simulink model "final_quadruped_210522"  (R2021a)
settings: Solver=ode15s  StartTime=0.0  StopTime=2  RelTol=1e-6  EnableMultiTasking=on
values from neighbouring files (symbols this model uses):
  foot_x = 8    [bipedparameters.m]    (also in fcn.m; finalrobotParameters.m; finalrobotParameters_110522.m; finalrobotParameters_140522.m)
  foot_y = 6    [bipedparameters.m]    (also in fcn.m; finalrobotParameters.m; finalrobotParameters_110522.m; finalrobotParameters_140522.m)
  foot_z = 1    [bipedparameters.m]    (also in fcn.m; finalrobotParameters.m; finalrobotParameters_110522.m; finalrobotParameters_140522.m)
  height_plane = 0.025    [bipedparameters.m]    (also in finalrobotParameters.m; finalrobotParameters_110522.m; finalrobotParameters_140522.m; finalrobotParameters_240522.m)
  kd = 1000    [bipedparameters.m]    (also in finalrobotParameters_140522.m = 5; finalrobotParameters_240522.m)
  ki = 1000    [bipedparameters.m]    (also in finalrobotParameters_140522.m = 5; finalrobotParameters_240522.m)
  kp = 1000    [bipedparameters.m]    (also in finalrobotParameters_140522.m = 5; finalrobotParameters_240522.m)
  lower_leg_length = 10    [bipedparameters.m]    (also in fcn.m; finalrobotParameters.m; finalrobotParameters_110522.m; finalrobotParameters_140522.m)
  m_ll = density*leg_radius*leg_radius*lower_leg_length*3.141592653589*0.01*0.01*0.01    (= 0.0176714586764)    [bipedparameters.m]    (also in fcn.m; finalrobotParameters_140522.m; finalrobotParameters_240522.m; hdotlb.m)
  m_ul = density*leg_radius*leg_radius*upper_leg_length*3.141592653589*0.01*0.01*0.01    (= 0.0176714586764)    [bipedparameters.m]    (also in fcn.m; finalrobotParameters_140522.m; finalrobotParameters_240522.m; hdotlb.m)
  plane_x = 25    [bipedparameters.m]    (also in finalrobotParameters.m; finalrobotParameters_110522.m; finalrobotParameters_140522.m; finalrobotParameters_240522.m)
  plane_y = 3    [bipedparameters.m]    (also in finalrobotParameters.m; finalrobotParameters_110522.m; finalrobotParameters_140522.m; finalrobotParameters_240522.m)
  torso_offset_x = -0.5    [bipedparameters.m]    (also in finalrobotParameters.m = 10; finalrobotParameters_110522.m = 10; finalrobotParameters_140522.m = 10; finalrobotParameters_240522.m = 10)
  torso_offset_z = -2    [bipedparameters.m]    (also in finalrobotParameters.m; finalrobotParameters_110522.m; finalrobotParameters_140522.m; finalrobotParameters_240522.m)
  torso_x = 5    [bipedparameters.m]    (also in fcn.m = 25; finalrobotParameters.m = 25; finalrobotParameters_110522.m = 25; finalrobotParameters_140522.m = 25)
  torso_y = 10    [bipedparameters.m]    (also in fcn.m = 16; finalrobotParameters.m = 16; finalrobotParameters_110522.m = 16; finalrobotParameters_140522.m = 16)
  torso_z = 8    [bipedparameters.m]    (also in fcn.m = 10; finalrobotParameters.m = 10; finalrobotParameters_110522.m = 10; finalrobotParameters_140522.m = 10)
  upper_leg_length = 10    [bipedparameters.m]    (also in fcn.m; finalrobotParameters.m; finalrobotParameters_110522.m; finalrobotParameters_140522.m)
undefined symbols (not defined in the file or in its folder): X, Y, Z
libraries: nesl_utility x151, sm_lib x71, Contact_Forces_Lib x16, pid_lib x12, fl_lib x4
(part 6 of 7)

== system final_quadruped_210522/Model/Right Leg Back/Knee ==
  note: accelerationRBknee
  note: Meas for knee
  tddRB_knee : Inport
  t2ddknee : Inport  Port=2
  Bus Creator : BusCreator  Inputs=3
  Knee joint : sm_lib/Joints/Revolute Joint  JointMode=Normal  SenseConstraintForce=off  SenseConstraintForceX=off  SenseConstraintForceY=off  SenseConstraintForceZ=off  SenseConstraintTorque=off  SenseConstraintTorqueX=off  SenseConstraintTorqueY=off  SenseConstraintTorqueZ=off  SenseTotalForce=off  SenseTotalForceX=off  SenseTotalForceY=off  SenseTotalForceZ=off  SenseTotalTorque=off  SenseTotalTorqueX=off  SenseTotalTorqueY=off  SenseTotalTorqueZ=off  CompositeWrenchDir=FollowerOnBase  CompositeWrenchFrame=BaseFrame  EquilibriumPosition=0  EquilibriumPositionUnits=deg  SpringStiffness=0  SpringStiffnessUnits=N*m/deg  DampingCoefficient=0  DampingCoefficientUnits=N*m/(deg/s)  TorqueActuationMode=InputTorque  MotionActuationMode=ComputedMotion  SensePosition=on  SenseVelocity=on  SenseAcceleration=on  SenseTorqueForce=off  SenseLowerLimitTorqueForce=off  SenseUpperLimitTorqueForce=off  LowerLimitSpecify=on  LowerLimitBound=0  LowerLimitBoundUnits=deg  LowerLimitStiffness=1e4  LowerLimitStiffnessUnits=N*m/deg  LowerLimitDamping=10  LowerLimitDampingUnits=N*m/(deg/s)  LowerLimitTransitionRegionWidth=0.1  LowerLimitTransitionRegionWidthUnits=deg  UpperLimitSpecify=on  UpperLimitBound=20  UpperLimitBoundUnits=deg  UpperLimitStiffness=1e4  UpperLimitStiffnessUnits=N*m/deg  UpperLimitDamping=10  UpperLimitDampingUnits=N*m/(deg/s)  UpperLimitTransitionRegionWidth=0.1  UpperLimitTransitionRegionWidthUnits=deg  PositionTargetSpecify=off  PositionTargetPriority=High  PositionTargetValue=0  PositionTargetValueUnits=deg  VelocityTargetSpecify=off  VelocityTargetPriority=High  VelocityTargetValue=0  VelocityTargetValueUnits=deg/s
  PID Controller : pid_lib/PID Controller  Controller=PID  Form=Parallel  TimeDomain=Continuous-time  UseExternalTs=off  SampleTime=-1  IntegratorMethod=Forward Euler  FilterMethod=Forward Euler  ControllerParametersSource=internal  P=kp  I=ki  D=kd  UseFilter=on  N=100  TunerSelectOption=Transfer Function Based (PID Tuner App)  InitialConditionSource=internal  InitialConditionForIntegrator=0  InitialConditionForFilter=0  DifferentiatorICPrevScaledInput=0  ExternalReset=none  TrackingMode=off  Kt=1  LimitOutput=off  SatLimitsSource=internal  UpperSaturationLimit=inf  LowerSaturationLimit=-inf  LinearizeAsGain=on  AntiWindupMode=none  Kb=1  POutMin=[]  POutMax=[]  IOutMin=[]  IOutMax=[]  DOutMin=[]  DOutMax=[]  NOutMin=[]  NOutMax=[]  SumOutMin=[]  SumOutMax=[]  SaturationOutMin=[]  SaturationOutMax=[]  PParamMin=[]  PParamMax=[]  IParamMin=[]  IParamMax=[]  DParamMin=[]  DParamMax=[]  NParamMin=[]  NParamMax=[]  KbParamMin=[]  KbParamMax=[]  KtParamMin=[]  KtParamMax=[]  KbOutMin=[]  KbOutMax=[]  KtOutMin=[]  KtOutMax=[]  IntegratorOutMin=[]  IntegratorOutMax=[]  FilterOutMin=[]  FilterOutMax=[]  SumI1OutMin=[]  SumI1OutMax=[]  SumI2OutMin=[]  SumI2OutMax=[]  SumI3OutMin=[]  SumI3OutMax=[]  SumI4OutMin=[]  SumI4OutMax=[]  SumDOutMin=[]  SumDOutMax=[]  DifferentiatorOutMin=[]  DifferentiatorOutMax=[]  FilterDiffOutCoefMin=[]  FilterDiffOutCoefMax=[]  ReciprocalOutMin=[]  ReciprocalOutMax=[]  SumDenOutMin=[]  SumDenOutMax=[]  SumNumOutMin=[]  SumNumOutMax=[]  DivideOutMin=[]  DivideOutMax=[]  UdiffTsProdOutMin=[]  UdiffTsProdOutMax=[]  NTsProdOutMin=[]  NTsProdOutMax=[]  UintegralTsProdOutMin=[]  UintegralTsProdOutMax=[]  UngainTsProdOutMin=[]  UngainTsProdOutMax=[]  IntegratorContinuousStateAttributes=''  IntegratorStateMustResolveToSignalObject=off  IntegratorRTWStateStorageClass=Auto  FilterContinuousStateAttributes=''  FilterStateMustResolveToSignalObject=off  FilterRTWStateStorageClass=Auto  ParallelPVariant=InternalParameters  IdealPVariant=Disabled  IVariant=InternalParameters  DVariant=InternalParameters  IntegratorVariant=Continuous  SatVariant=Disabled  AWVariant=Passthrough  PCopyVariant=Disabled  TRVariant=Disabled  FdbkBlocksVariant=Forward  IdealPFdbkVariant=Disabled  SatFdbkVariant=Disabled  DerivativeFilterVariant=ContFilter  NVariant=InternalParameters  NCopyVariant=Disabled  FilterICVariant=InternalICsFilter  IntegratorICVariant=InternalICs  ExternalResetVariant=Disabled  TRSumVariant=Passthrough  SumFdbkVariant=Disabled  SumVariant=Sum_PID  TsampFilterVariant=InternalTs  TsampNgainVariant=Passthrough  TsampIntegralVariant=Passthrough  ExternalSaturationOutDataTypeStr=Inherit: Same as second input
  PS-Simulink Converter : nesl_utility/PS-Simulink Converter  PhysicalDomain=network_engine_domain  SubClassName=ps_output  LeftPortType=input  RightPortType=output  PseudoPeriodic=off  Frequencies=[]  Unit=inherit  AffineConversion=off
      settings: SourceProductBaseCode=PW,SS
  PS-Simulink Converter1 : nesl_utility/PS-Simulink Converter  PhysicalDomain=network_engine_domain  SubClassName=ps_output  LeftPortType=input  RightPortType=output  PseudoPeriodic=off  Frequencies=[]  Unit=1  AffineConversion=off
      settings: SourceProductBaseCode=PW,SS
  PS-Simulink Converter3 : nesl_utility/PS-Simulink Converter  PhysicalDomain=network_engine_domain  SubClassName=ps_output  LeftPortType=input  RightPortType=output  PseudoPeriodic=off  Frequencies=[]  Unit=1  AffineConversion=off
      settings: SourceProductBaseCode=PW,SS
  Scope : Scope
  Scope1 : Scope
  Scope2 : Scope
  Simulink-PS Converter : nesl_utility/Simulink-PS Converter  PhysicalDomain=network_engine_domain  SubClassName=ps_input  LeftPortType=input  RightPortType=output  PseudoPeriodic=off  Frequencies=[]  NoiseDistribution=none  NoiseParameters=[]  Unit=1  AffineConversion=off  FilteringAndDerivatives=provide  SimscapeFilterOrder=1  InputFilterTimeConstant=0.001  UdotUserProvided=0
      settings: SourceProductBaseCode=PW,SS
  Sum : Sum  Inputs=|+-
  Conn1 : PMIOPort  Side=Left
  Conn2 : PMIOPort  Port=2  Side=Right
  q : PMIOPort  Port=3  Side=Left
  meas : Outport
  Outport : Outport  Port=2
  Outport1 : Outport  Port=3
  wires:
  Bus Creator/1 -> meas/1
  PS-Simulink Converter3/1 -> Bus Creator/1  "angleRBknee"
  Sum/1 -> Scope/1, PID Controller/1
  PS-Simulink Converter1/1 -> Outport/1, Bus Creator/2  "speedRBknee"
  PID Controller/1 -> Bus Creator/3, Simulink-PS Converter/1, Scope1/1  "torqueRBknee"
  tddRB_knee/1 -> Scope2/1
  t2ddknee/1 -> Sum/1
  PS-Simulink Converter/1 -> Outport1/1, Sum/2
  connections:
  Conn2/RConn1 -- Knee joint/RConn1
  q/RConn1 -- PS-Simulink Converter3/LConn1 -- Knee joint/RConn2
  Knee joint/LConn1 -- Conn1/RConn1
  Knee joint/RConn3 -- PS-Simulink Converter1/LConn1
  Simulink-PS Converter/RConn1 -- Knee joint/LConn2
  Knee joint/RConn4 -- PS-Simulink Converter/LConn1

== system final_quadruped_210522/Model/Right Leg Back/Measuring Component ==
  Fn : Inport
  Hip : Inport  Port=2
  Fr : Inport  Port=3
  Knee : Inport  Port=4
  Ankle : Inport  Port=5
  Bus Creator : BusCreator  Inputs=9
  Bus Selector : BusSelector  OutputSignals=angleRBknee,speedRBknee,torqueRBknee
  Bus Selector1 : BusSelector  OutputSignals=angleRBhip,speedRBhip,torqueRBhip
  Meas : Outport  VectorParamsAs1DForOutWhenUnconnected=off
  wires:
  Ankle/1 -> Bus Creator/3
  Bus Selector1/2 -> Bus Creator/8  "<speedRBhip>"
  Hip/1 -> Bus Selector1/1
  Fn/1 -> Bus Creator/1
  Bus Selector/3 -> Bus Creator/6  "<torqueRBknee>"
  Bus Creator/1 -> Meas/1
  Fr/1 -> Bus Creator/2
  Knee/1 -> Bus Selector/1
  Bus Selector1/3 -> Bus Creator/9  "<torqueRBhip>"
  Bus Selector/2 -> Bus Creator/5  "<speedRBknee>"
  Bus Selector/1 -> Bus Creator/4  "<angleRBknee>"
  Bus Selector1/1 -> Bus Creator/7  "<angleRBhip>"

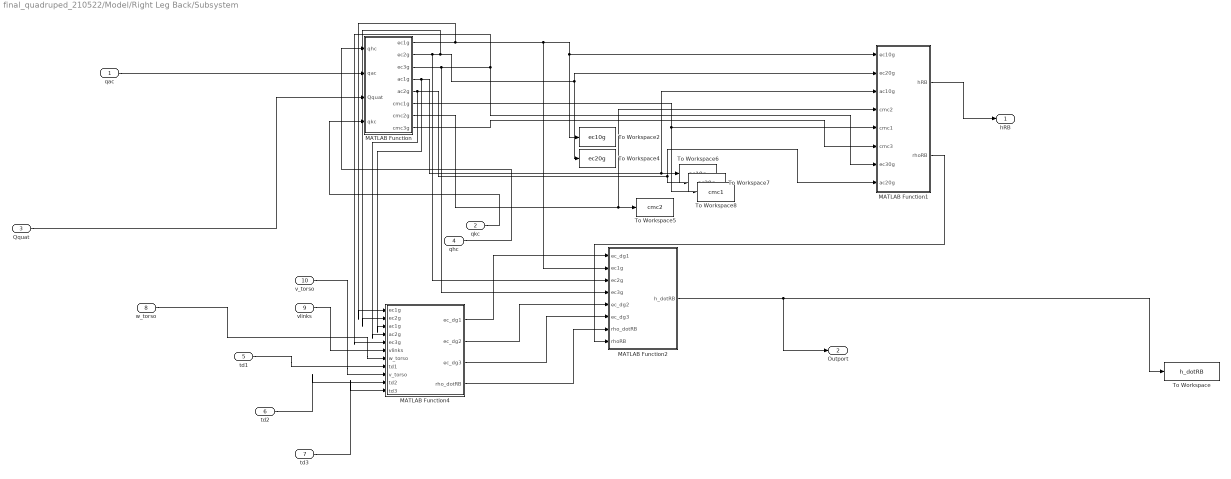
== system final_quadruped_210522/Model/Right Leg Back/Subsystem ==
  qac : Inport
  qkc : Inport  Port=2
  Qquat : Inport  Port=3
  qhc : Inport  Port=4
  td1 : Inport  Port=5
  td2 : Inport  Port=6
  td3 : Inport  Port=7
  w_torso : Inport  Port=8
  vlinks : Inport  Port=9
  v_torso : Inport  Port=10
  MATLAB Function : MATLAB Function  TreatAsAtomicUnit=on
  MATLAB Function1 : MATLAB Function  TreatAsAtomicUnit=on
  MATLAB Function2 : MATLAB Function  TreatAsAtomicUnit=on
  MATLAB Function4 : MATLAB Function  TreatAsAtomicUnit=on
  To Workspace : ToWorkspace  VariableName=h_dotRB  SaveFormat=Timeseries  SampleTime=-1
  To Workspace2 : ToWorkspace  VariableName=ec10g  SaveFormat=Timeseries  SampleTime=-1
  To Workspace4 : ToWorkspace  VariableName=ec20g  SaveFormat=Timeseries  SampleTime=-1
  To Workspace5 : ToWorkspace  VariableName=cmc2  SaveFormat=Timeseries  SampleTime=-1
  To Workspace6 : ToWorkspace  VariableName=ac10g  SaveFormat=Timeseries  SampleTime=-1
  To Workspace7 : ToWorkspace  VariableName=ac20g  SaveFormat=Timeseries  SampleTime=-1
  To Workspace8 : ToWorkspace  VariableName=cmc1  SaveFormat=Timeseries  SampleTime=-1
  hRB : Outport
  Outport : Outport  Port=2
  wires:
  MATLAB Function/6(cmc1g) -> To Workspace8/1, MATLAB Function1/5(cmc1)
  MATLAB Function/5(ac2g) -> MATLAB Function4/4(ac2g), To Workspace7/1, MATLAB Function1/8(ac20g)
  MATLAB Function/1(ec1g) -> To Workspace2/1, MATLAB Function1/1(ec10g), MATLAB Function2/2(ec1g), MATLAB Function4/1(ec1g)
  MATLAB Function/8(cmc3g) -> MATLAB Function1/6(cmc3)
  qac/1 -> MATLAB Function/2(qac)
  MATLAB Function/7(cmc2g) -> MATLAB Function1/4(cmc2), To Workspace5/1
  MATLAB Function/4(ac1g) -> MATLAB Function4/3(ac1g), To Workspace6/1, MATLAB Function1/3(ac10g)
  MATLAB Function/3(ec3g) -> MATLAB Function2/4(ec3g), MATLAB Function1/7(ec30g), MATLAB Function4/5(ec3g)
  MATLAB Function/2(ec2g) -> MATLAB Function2/3(ec2g), MATLAB Function4/2(ec2g), To Workspace4/1, MATLAB Function1/2(ec20g)
  qhc/1 -> MATLAB Function/1(qhc)
  Qquat/1 -> MATLAB Function/3(Qquat)
  MATLAB Function1/1(hRB) -> hRB/1
  qkc/1 -> MATLAB Function/4(qkc)
  td2/1 -> MATLAB Function4/10(td2)
  v_torso/1 -> MATLAB Function4/9(v_torso)
  MATLAB Function4/4(rho_dotRB) -> MATLAB Function2/7(rho_dotRB)
  MATLAB Function4/1(ec_dg1) -> MATLAB Function2/1(ec_dg1)
  vlinks/1 -> MATLAB Function4/6(vlinks)
  MATLAB Function2/1(h_dotRB) -> Outport/1, To Workspace/1
  td3/1 -> MATLAB Function4/11(td3)
  MATLAB Function4/3(ec_dg3) -> MATLAB Function2/6(ec_dg3)
  td1/1 -> MATLAB Function4/8(td1)
  MATLAB Function4/2(ec_dg2) -> MATLAB Function2/5(ec_dg2)
  MATLAB Function1/2(rhoRB) -> MATLAB Function2/8(rhoRB)
  w_torso/1 -> MATLAB Function4/7(w_torso)

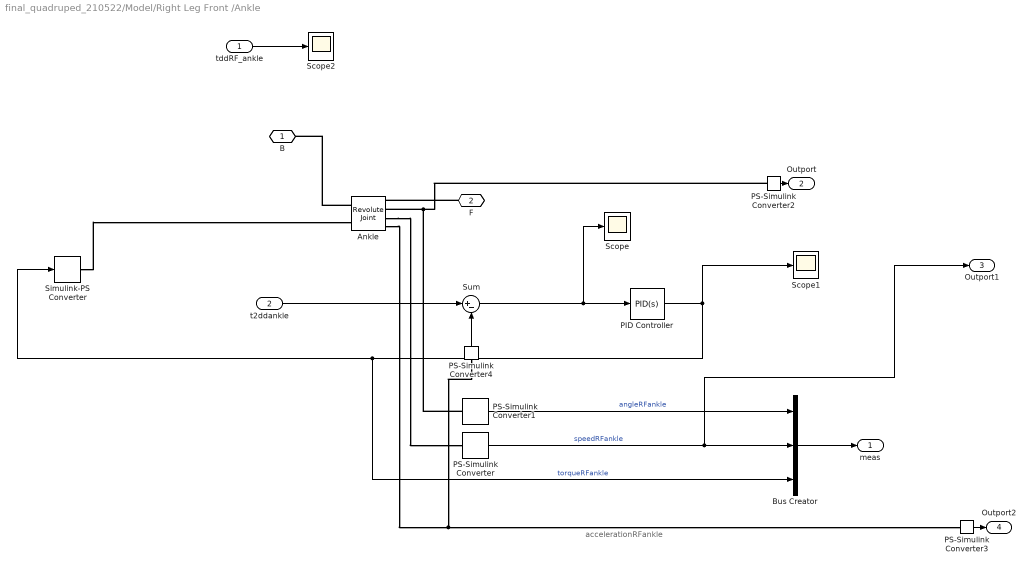
== system final_quadruped_210522/Model/Right Leg Front /Ankle  ==
  note: accelerationRFankle
  tddRF_ankle : Inport
  t2ddankle : Inport  Port=2
  Ankle : sm_lib/Joints/Revolute Joint  JointMode=Normal  SenseConstraintForce=off  SenseConstraintForceX=off  SenseConstraintForceY=off  SenseConstraintForceZ=off  SenseConstraintTorque=off  SenseConstraintTorqueX=off  SenseConstraintTorqueY=off  SenseConstraintTorqueZ=off  SenseTotalForce=off  SenseTotalForceX=off  SenseTotalForceY=off  SenseTotalForceZ=off  SenseTotalTorque=off  SenseTotalTorqueX=off  SenseTotalTorqueY=off  SenseTotalTorqueZ=off  CompositeWrenchDir=FollowerOnBase  CompositeWrenchFrame=BaseFrame  EquilibriumPosition=0  EquilibriumPositionUnits=deg  SpringStiffness=0  SpringStiffnessUnits=N*m/deg  DampingCoefficient=0  DampingCoefficientUnits=N*m/(deg/s)  TorqueActuationMode=InputTorque  MotionActuationMode=ComputedMotion  SensePosition=on  SenseVelocity=on  SenseAcceleration=on  SenseTorqueForce=off  SenseLowerLimitTorqueForce=off  SenseUpperLimitTorqueForce=off  LowerLimitSpecify=off  LowerLimitBound=-90  LowerLimitBoundUnits=deg  LowerLimitStiffness=1e4  LowerLimitStiffnessUnits=N*m/deg  LowerLimitDamping=10  LowerLimitDampingUnits=N*m/(deg/s)  LowerLimitTransitionRegionWidth=0.1  LowerLimitTransitionRegionWidthUnits=deg  UpperLimitSpecify=off  UpperLimitBound=90  UpperLimitBoundUnits=deg  UpperLimitStiffness=1e4  UpperLimitStiffnessUnits=N*m/deg  UpperLimitDamping=10  UpperLimitDampingUnits=N*m/(deg/s)  UpperLimitTransitionRegionWidth=0.1  UpperLimitTransitionRegionWidthUnits=deg  PositionTargetSpecify=off  PositionTargetPriority=High  PositionTargetValue=0  PositionTargetValueUnits=deg  VelocityTargetSpecify=off  VelocityTargetPriority=High  VelocityTargetValue=0  VelocityTargetValueUnits=deg/s
  Bus Creator : BusCreator  Inputs=3
  PID Controller : pid_lib/PID Controller  Controller=PID  Form=Parallel  TimeDomain=Continuous-time  UseExternalTs=off  SampleTime=-1  IntegratorMethod=Forward Euler  FilterMethod=Forward Euler  ControllerParametersSource=internal  P=kp  I=ki  D=kd  UseFilter=on  N=100  TunerSelectOption=Transfer Function Based (PID Tuner App)  InitialConditionSource=internal  InitialConditionForIntegrator=0  InitialConditionForFilter=0  DifferentiatorICPrevScaledInput=0  ExternalReset=none  TrackingMode=off  Kt=1  LimitOutput=off  SatLimitsSource=internal  UpperSaturationLimit=inf  LowerSaturationLimit=-inf  LinearizeAsGain=on  AntiWindupMode=none  Kb=1  POutMin=[]  POutMax=[]  IOutMin=[]  IOutMax=[]  DOutMin=[]  DOutMax=[]  NOutMin=[]  NOutMax=[]  SumOutMin=[]  SumOutMax=[]  SaturationOutMin=[]  SaturationOutMax=[]  PParamMin=[]  PParamMax=[]  IParamMin=[]  IParamMax=[]  DParamMin=[]  DParamMax=[]  NParamMin=[]  NParamMax=[]  KbParamMin=[]  KbParamMax=[]  KtParamMin=[]  KtParamMax=[]  KbOutMin=[]  KbOutMax=[]  KtOutMin=[]  KtOutMax=[]  IntegratorOutMin=[]  IntegratorOutMax=[]  FilterOutMin=[]  FilterOutMax=[]  SumI1OutMin=[]  SumI1OutMax=[]  SumI2OutMin=[]  SumI2OutMax=[]  SumI3OutMin=[]  SumI3OutMax=[]  SumI4OutMin=[]  SumI4OutMax=[]  SumDOutMin=[]  SumDOutMax=[]  DifferentiatorOutMin=[]  DifferentiatorOutMax=[]  FilterDiffOutCoefMin=[]  FilterDiffOutCoefMax=[]  ReciprocalOutMin=[]  ReciprocalOutMax=[]  SumDenOutMin=[]  SumDenOutMax=[]  SumNumOutMin=[]  SumNumOutMax=[]  DivideOutMin=[]  DivideOutMax=[]  UdiffTsProdOutMin=[]  UdiffTsProdOutMax=[]  NTsProdOutMin=[]  NTsProdOutMax=[]  UintegralTsProdOutMin=[]  UintegralTsProdOutMax=[]  UngainTsProdOutMin=[]  UngainTsProdOutMax=[]  IntegratorContinuousStateAttributes=''  IntegratorStateMustResolveToSignalObject=off  IntegratorRTWStateStorageClass=Auto  FilterContinuousStateAttributes=''  FilterStateMustResolveToSignalObject=off  FilterRTWStateStorageClass=Auto  ParallelPVariant=InternalParameters  IdealPVariant=Disabled  IVariant=InternalParameters  DVariant=InternalParameters  IntegratorVariant=Continuous  SatVariant=Disabled  AWVariant=Passthrough  PCopyVariant=Disabled  TRVariant=Disabled  FdbkBlocksVariant=Forward  IdealPFdbkVariant=Disabled  SatFdbkVariant=Disabled  DerivativeFilterVariant=ContFilter  NVariant=InternalParameters  NCopyVariant=Disabled  FilterICVariant=InternalICsFilter  IntegratorICVariant=InternalICs  ExternalResetVariant=Disabled  TRSumVariant=Passthrough  SumFdbkVariant=Disabled  SumVariant=Sum_PID  TsampFilterVariant=InternalTs  TsampNgainVariant=Passthrough  TsampIntegralVariant=Passthrough  ExternalSaturationOutDataTypeStr=Inherit: Same as second input
  PS-Simulink Converter : nesl_utility/PS-Simulink Converter  PhysicalDomain=network_engine_domain  SubClassName=ps_output  LeftPortType=input  RightPortType=output  PseudoPeriodic=off  Frequencies=[]  Unit=1  AffineConversion=off
      settings: SourceProductBaseCode=PW,SS
  PS-Simulink Converter1 : nesl_utility/PS-Simulink Converter  PhysicalDomain=network_engine_domain  SubClassName=ps_output  LeftPortType=input  RightPortType=output  PseudoPeriodic=off  Frequencies=[]  Unit=1  AffineConversion=off
      settings: SourceProductBaseCode=PW,SS
  PS-Simulink Converter2 : nesl_utility/PS-Simulink Converter  PhysicalDomain=network_engine_domain  SubClassName=ps_output  LeftPortType=input  RightPortType=output  PseudoPeriodic=off  Frequencies=[]  Unit=inherit  AffineConversion=off
      settings: SourceProductBaseCode=PW,SS
  PS-Simulink Converter3 : nesl_utility/PS-Simulink Converter  PhysicalDomain=network_engine_domain  SubClassName=ps_output  LeftPortType=input  RightPortType=output  PseudoPeriodic=off  Frequencies=[]  Unit=inherit  AffineConversion=off
      settings: SourceProductBaseCode=PW,SS
  PS-Simulink Converter4 : nesl_utility/PS-Simulink Converter  PhysicalDomain=network_engine_domain  SubClassName=ps_output  LeftPortType=input  RightPortType=output  PseudoPeriodic=off  Frequencies=[]  Unit=inherit  AffineConversion=off
      settings: SourceProductBaseCode=PW,SS
  Scope : Scope
  Scope1 : Scope
  Scope2 : Scope
  Simulink-PS Converter : nesl_utility/Simulink-PS Converter  PhysicalDomain=network_engine_domain  SubClassName=ps_input  LeftPortType=input  RightPortType=output  PseudoPeriodic=off  Frequencies=[]  NoiseDistribution=none  NoiseParameters=[]  Unit=1  AffineConversion=off  FilteringAndDerivatives=provide  SimscapeFilterOrder=1  InputFilterTimeConstant=0.001  UdotUserProvided=0
      settings: SourceProductBaseCode=PW,SS
  Sum : Sum  Inputs=|+-
  B : PMIOPort  Side=Left
  F : PMIOPort  Port=2  Side=Right
  meas : Outport  VectorParamsAs1DForOutWhenUnconnected=off
  Outport : Outport  Port=2
  Outport1 : Outport  Port=3
  Outport2 : Outport  Port=4
  wires:
  PS-Simulink Converter1/1 -> Bus Creator/1  "angleRFankle"
  PS-Simulink Converter/1 -> Outport1/1, Bus Creator/2  "speedRFankle"
  PID Controller/1 -> Scope1/1, Simulink-PS Converter/1, Bus Creator/3  "torqueRFankle"
  Bus Creator/1 -> meas/1
  Sum/1 -> PID Controller/1, Scope/1
  PS-Simulink Converter2/1 -> Outport/1
  PS-Simulink Converter3/1 -> Outport2/1
  t2ddankle/1 -> Sum/1
  PS-Simulink Converter4/1 -> Sum/2
  tddRF_ankle/1 -> Scope2/1
  connections:
  F/RConn1 -- Ankle/RConn1
  Ankle/LConn1 -- B/RConn1
  PS-Simulink Converter1/LConn1 -- Ankle/RConn2 -- PS-Simulink Converter2/LConn1
  Ankle/RConn3 -- PS-Simulink Converter/LConn1
  Simulink-PS Converter/RConn1 -- Ankle/LConn2
  Ankle/RConn4 -- PS-Simulink Converter3/LConn1 -- PS-Simulink Converter4/LConn1

== system final_quadruped_210522/Model/Right Leg Front /Contact Forces  ==
  In1 : Inport
  In2 : Inport  Port=2
  In3 : Inport  Port=3
  Qd3g : Inport  Port=4
  In4 : Inport  Port=5
  Add : Sum  Inputs=++++
  Add1 : Sum  Inputs=++++
  Bus Selector{,1..3} (4 alike) : BusSelector  OutputSignals=Normal Force,Friction Force
  MATLAB Function : MATLAB Function  TreatAsAtomicUnit=on
  Math Function : Math  Operator=square  SignedPower=on  SaturateOnIntegerOverflow=on
  Scope : Scope
  Scope1 : Scope
  Sqrt : Sqrt  SaturateOnIntegerOverflow=on
  Sum of Elements : Sum  Inputs=+
  Out1 : Outport  VectorParamsAs1DForOutWhenUnconnected=off
  Out2 : Outport  Port=2  VectorParamsAs1DForOutWhenUnconnected=off
  Outport : Outport  Port=3
  Outport1 : Outport  Port=4
  wires:
  Sqrt/1 -> Out2/1
  Add/1 -> Out1/1
  Sum of Elements/1 -> Sqrt/1
  Bus Selector1/2 -> Add1/2, MATLAB Function/6(f2)  "<Friction Force>"
  Bus Selector2/1 -> MATLAB Function/4(n3), Add/3  "<Normal Force>"
  Bus Selector3/2 -> Scope1/1, MATLAB Function/8(f4), Add1/4  "<Friction Force>"
  Bus Selector3/1 -> Add/4, MATLAB Function/3(n4)  "<Normal Force>"
  Bus Selector/1 -> Add/1, Scope/1, MATLAB Function/1(n1)  "<Normal Force>"
  Bus Selector/2 -> MATLAB Function/5(f1), Add1/1  "<Friction Force>"
  Bus Selector1/1 -> Add/2, MATLAB Function/2(n2)  "<Normal Force>"
  In3/1 -> Bus Selector2/1
  Add1/1 -> Math Function/1
  Math Function/1 -> Sum of Elements/1
  In2/1 -> Bus Selector1/1
  Bus Selector2/2 -> MATLAB Function/7(f3), Add1/3  "<Friction Force>"
  In1/1 -> Bus Selector/1
  In4/1 -> Bus Selector3/1
  MATLAB Function/1(NRF) -> Outport/1
  MATLAB Function/2(FRF) -> Outport1/1
  Qd3g/1 -> MATLAB Function/9(Qd3g)

== system final_quadruped_210522/Model/Right Leg Front /Hip ==
  note: accelerationRFhip
  note: Meas for hip
  t2ddhip : Inport
  tddRF_hip : Inport  Port=2
  Bus Creator : BusCreator  Inputs=3
  Hip joint : sm_lib/Joints/Revolute Joint  JointMode=Normal  SenseConstraintForce=off  SenseConstraintForceX=off  SenseConstraintForceY=off  SenseConstraintForceZ=off  SenseConstraintTorque=off  SenseConstraintTorqueX=off  SenseConstraintTorqueY=off  SenseConstraintTorqueZ=off  SenseTotalForce=off  SenseTotalForceX=off  SenseTotalForceY=off  SenseTotalForceZ=off  SenseTotalTorque=off  SenseTotalTorqueX=off  SenseTotalTorqueY=off  SenseTotalTorqueZ=off  CompositeWrenchDir=FollowerOnBase  CompositeWrenchFrame=BaseFrame  EquilibriumPosition=0  EquilibriumPositionUnits=deg  SpringStiffness=0  SpringStiffnessUnits=N*m/deg  DampingCoefficient=0  DampingCoefficientUnits=N*m/(deg/s)  TorqueActuationMode=InputTorque  MotionActuationMode=ComputedMotion  SensePosition=on  SenseVelocity=on  SenseAcceleration=on  SenseTorqueForce=off  SenseLowerLimitTorqueForce=off  SenseUpperLimitTorqueForce=off  LowerLimitSpecify=on  LowerLimitBound=0  LowerLimitBoundUnits=deg  LowerLimitStiffness=1e4  LowerLimitStiffnessUnits=N*m/deg  LowerLimitDamping=10  LowerLimitDampingUnits=N*m/(deg/s)  LowerLimitTransitionRegionWidth=0.1  LowerLimitTransitionRegionWidthUnits=deg  UpperLimitSpecify=on  UpperLimitBound=20  UpperLimitBoundUnits=deg  UpperLimitStiffness=1e4  UpperLimitStiffnessUnits=N*m/deg  UpperLimitDamping=10  UpperLimitDampingUnits=N*m/(deg/s)  UpperLimitTransitionRegionWidth=0.1  UpperLimitTransitionRegionWidthUnits=deg  PositionTargetSpecify=off  PositionTargetPriority=High  PositionTargetValue=0  PositionTargetValueUnits=deg  VelocityTargetSpecify=off  VelocityTargetPriority=High  VelocityTargetValue=0  VelocityTargetValueUnits=deg/s
  PID Controller : pid_lib/PID Controller  Controller=PID  Form=Parallel  TimeDomain=Continuous-time  UseExternalTs=off  SampleTime=-1  IntegratorMethod=Forward Euler  FilterMethod=Forward Euler  ControllerParametersSource=internal  P=kp  I=ki  D=kd  UseFilter=on  N=100  TunerSelectOption=Transfer Function Based (PID Tuner App)  InitialConditionSource=internal  InitialConditionForIntegrator=0  InitialConditionForFilter=0  DifferentiatorICPrevScaledInput=0  ExternalReset=none  TrackingMode=off  Kt=1  LimitOutput=off  SatLimitsSource=internal  UpperSaturationLimit=inf  LowerSaturationLimit=-inf  LinearizeAsGain=on  AntiWindupMode=none  Kb=1  POutMin=[]  POutMax=[]  IOutMin=[]  IOutMax=[]  DOutMin=[]  DOutMax=[]  NOutMin=[]  NOutMax=[]  SumOutMin=[]  SumOutMax=[]  SaturationOutMin=[]  SaturationOutMax=[]  PParamMin=[]  PParamMax=[]  IParamMin=[]  IParamMax=[]  DParamMin=[]  DParamMax=[]  NParamMin=[]  NParamMax=[]  KbParamMin=[]  KbParamMax=[]  KtParamMin=[]  KtParamMax=[]  KbOutMin=[]  KbOutMax=[]  KtOutMin=[]  KtOutMax=[]  IntegratorOutMin=[]  IntegratorOutMax=[]  FilterOutMin=[]  FilterOutMax=[]  SumI1OutMin=[]  SumI1OutMax=[]  SumI2OutMin=[]  SumI2OutMax=[]  SumI3OutMin=[]  SumI3OutMax=[]  SumI4OutMin=[]  SumI4OutMax=[]  SumDOutMin=[]  SumDOutMax=[]  DifferentiatorOutMin=[]  DifferentiatorOutMax=[]  FilterDiffOutCoefMin=[]  FilterDiffOutCoefMax=[]  ReciprocalOutMin=[]  ReciprocalOutMax=[]  SumDenOutMin=[]  SumDenOutMax=[]  SumNumOutMin=[]  SumNumOutMax=[]  DivideOutMin=[]  DivideOutMax=[]  UdiffTsProdOutMin=[]  UdiffTsProdOutMax=[]  NTsProdOutMin=[]  NTsProdOutMax=[]  UintegralTsProdOutMin=[]  UintegralTsProdOutMax=[]  UngainTsProdOutMin=[]  UngainTsProdOutMax=[]  IntegratorContinuousStateAttributes=''  IntegratorStateMustResolveToSignalObject=off  IntegratorRTWStateStorageClass=Auto  FilterContinuousStateAttributes=''  FilterStateMustResolveToSignalObject=off  FilterRTWStateStorageClass=Auto  ParallelPVariant=InternalParameters  IdealPVariant=Disabled  IVariant=InternalParameters  DVariant=InternalParameters  IntegratorVariant=Continuous  SatVariant=Disabled  AWVariant=Passthrough  PCopyVariant=Disabled  TRVariant=Disabled  FdbkBlocksVariant=Forward  IdealPFdbkVariant=Disabled  SatFdbkVariant=Disabled  DerivativeFilterVariant=ContFilter  NVariant=InternalParameters  NCopyVariant=Disabled  FilterICVariant=InternalICsFilter  IntegratorICVariant=InternalICs  ExternalResetVariant=Disabled  TRSumVariant=Passthrough  SumFdbkVariant=Disabled  SumVariant=Sum_PID  TsampFilterVariant=InternalTs  TsampNgainVariant=Passthrough  TsampIntegralVariant=Passthrough  ExternalSaturationOutDataTypeStr=Inherit: Same as second input
  PS-Simulink Converter1 : nesl_utility/PS-Simulink Converter  PhysicalDomain=network_engine_domain  SubClassName=ps_output  LeftPortType=input  RightPortType=output  PseudoPeriodic=off  Frequencies=[]  Unit=1  AffineConversion=off
      settings: SourceProductBaseCode=PW,SS
  PS-Simulink Converter2 : nesl_utility/PS-Simulink Converter  PhysicalDomain=network_engine_domain  SubClassName=ps_output  LeftPortType=input  RightPortType=output  PseudoPeriodic=off  Frequencies=[]  Unit=inherit  AffineConversion=off
      settings: SourceProductBaseCode=PW,SS
  PS-Simulink Converter3 : nesl_utility/PS-Simulink Converter  PhysicalDomain=network_engine_domain  SubClassName=ps_output  LeftPortType=input  RightPortType=output  PseudoPeriodic=off  Frequencies=[]  Unit=1  AffineConversion=off
      settings: SourceProductBaseCode=PW,SS
  Scope : Scope
  Scope1 : Scope
  Scope2 : Scope
  Simulink-PS Converter : nesl_utility/Simulink-PS Converter  PhysicalDomain=network_engine_domain  SubClassName=ps_input  LeftPortType=input  RightPortType=output  PseudoPeriodic=off  Frequencies=[]  NoiseDistribution=none  NoiseParameters=[]  Unit=1  AffineConversion=off  FilteringAndDerivatives=provide  SimscapeFilterOrder=1  InputFilterTimeConstant=0.001  UdotUserProvided=0
      settings: SourceProductBaseCode=PW,SS
  Sum : Sum  Inputs=|+-
  Conn1 : PMIOPort  Side=Left
  Conn2 : PMIOPort  Port=2  Side=Right
  q : PMIOPort  Port=3  Side=Left
  meas : Outport
  Outport : Outport  Port=2
  Outport2 : Outport  Port=3
  wires:
  Bus Creator/1 -> meas/1
  PS-Simulink Converter3/1 -> Bus Creator/1  "angleRFhip"
  PS-Simulink Converter1/1 -> Outport/1, Bus Creator/2  "speedRFhip"
  Sum/1 -> PID Controller/1, Scope/1
  PID Controller/1 -> Scope1/1, Bus Creator/3, Simulink-PS Converter/1  "torqueRFhip"
  t2ddhip/1 -> Sum/1
  PS-Simulink Converter2/1 -> Sum/2, Outport2/1
  tddRF_hip/1 -> Scope2/1
  connections:
  Hip joint/RConn2 -- PS-Simulink Converter3/LConn1 -- q/RConn1
  Conn2/RConn1 -- Hip joint/RConn1
  Hip joint/LConn1 -- Conn1/RConn1
  Hip joint/RConn3 -- PS-Simulink Converter1/LConn1
  Simulink-PS Converter/RConn1 -- Hip joint/LConn2
  PS-Simulink Converter2/LConn1 -- Hip joint/RConn4

== system final_quadruped_210522/Model/Right Leg Front /Knee ==
  note: accelerationRFknee
  note: Meas for knee
  tddRF_knee : Inport
  t2ddknee : Inport  Port=2
  Bus Creator : BusCreator  Inputs=3
  Knee joint : sm_lib/Joints/Revolute Joint  JointMode=Normal  SenseConstraintForce=off  SenseConstraintForceX=off  SenseConstraintForceY=off  SenseConstraintForceZ=off  SenseConstraintTorque=off  SenseConstraintTorqueX=off  SenseConstraintTorqueY=off  SenseConstraintTorqueZ=off  SenseTotalForce=off  SenseTotalForceX=off  SenseTotalForceY=off  SenseTotalForceZ=off  SenseTotalTorque=off  SenseTotalTorqueX=off  SenseTotalTorqueY=off  SenseTotalTorqueZ=off  CompositeWrenchDir=FollowerOnBase  CompositeWrenchFrame=BaseFrame  EquilibriumPosition=0  EquilibriumPositionUnits=deg  SpringStiffness=0  SpringStiffnessUnits=N*m/deg  DampingCoefficient=0  DampingCoefficientUnits=N*m/(deg/s)  TorqueActuationMode=InputTorque  MotionActuationMode=ComputedMotion  SensePosition=on  SenseVelocity=on  SenseAcceleration=on  SenseTorqueForce=off  SenseLowerLimitTorqueForce=off  SenseUpperLimitTorqueForce=off  LowerLimitSpecify=on  LowerLimitBound=0  LowerLimitBoundUnits=deg  LowerLimitStiffness=1e4  LowerLimitStiffnessUnits=N*m/deg  LowerLimitDamping=10  LowerLimitDampingUnits=N*m/(deg/s)  LowerLimitTransitionRegionWidth=0.1  LowerLimitTransitionRegionWidthUnits=deg  UpperLimitSpecify=on  UpperLimitBound=20  UpperLimitBoundUnits=deg  UpperLimitStiffness=1e4  UpperLimitStiffnessUnits=N*m/deg  UpperLimitDamping=10  UpperLimitDampingUnits=N*m/(deg/s)  UpperLimitTransitionRegionWidth=0.1  UpperLimitTransitionRegionWidthUnits=deg  PositionTargetSpecify=off  PositionTargetPriority=High  PositionTargetValue=0  PositionTargetValueUnits=deg  VelocityTargetSpecify=off  VelocityTargetPriority=High  VelocityTargetValue=0  VelocityTargetValueUnits=deg/s
  PID Controller : pid_lib/PID Controller  Controller=PID  Form=Parallel  TimeDomain=Continuous-time  UseExternalTs=off  SampleTime=-1  IntegratorMethod=Forward Euler  FilterMethod=Forward Euler  ControllerParametersSource=internal  P=kp  I=ki  D=kd  UseFilter=on  N=100  TunerSelectOption=Transfer Function Based (PID Tuner App)  InitialConditionSource=internal  InitialConditionForIntegrator=0  InitialConditionForFilter=0  DifferentiatorICPrevScaledInput=0  ExternalReset=none  TrackingMode=off  Kt=1  LimitOutput=off  SatLimitsSource=internal  UpperSaturationLimit=inf  LowerSaturationLimit=-inf  LinearizeAsGain=on  AntiWindupMode=none  Kb=1  POutMin=[]  POutMax=[]  IOutMin=[]  IOutMax=[]  DOutMin=[]  DOutMax=[]  NOutMin=[]  NOutMax=[]  SumOutMin=[]  SumOutMax=[]  SaturationOutMin=[]  SaturationOutMax=[]  PParamMin=[]  PParamMax=[]  IParamMin=[]  IParamMax=[]  DParamMin=[]  DParamMax=[]  NParamMin=[]  NParamMax=[]  KbParamMin=[]  KbParamMax=[]  KtParamMin=[]  KtParamMax=[]  KbOutMin=[]  KbOutMax=[]  KtOutMin=[]  KtOutMax=[]  IntegratorOutMin=[]  IntegratorOutMax=[]  FilterOutMin=[]  FilterOutMax=[]  SumI1OutMin=[]  SumI1OutMax=[]  SumI2OutMin=[]  SumI2OutMax=[]  SumI3OutMin=[]  SumI3OutMax=[]  SumI4OutMin=[]  SumI4OutMax=[]  SumDOutMin=[]  SumDOutMax=[]  DifferentiatorOutMin=[]  DifferentiatorOutMax=[]  FilterDiffOutCoefMin=[]  FilterDiffOutCoefMax=[]  ReciprocalOutMin=[]  ReciprocalOutMax=[]  SumDenOutMin=[]  SumDenOutMax=[]  SumNumOutMin=[]  SumNumOutMax=[]  DivideOutMin=[]  DivideOutMax=[]  UdiffTsProdOutMin=[]  UdiffTsProdOutMax=[]  NTsProdOutMin=[]  NTsProdOutMax=[]  UintegralTsProdOutMin=[]  UintegralTsProdOutMax=[]  UngainTsProdOutMin=[]  UngainTsProdOutMax=[]  IntegratorContinuousStateAttributes=''  IntegratorStateMustResolveToSignalObject=off  IntegratorRTWStateStorageClass=Auto  FilterContinuousStateAttributes=''  FilterStateMustResolveToSignalObject=off  FilterRTWStateStorageClass=Auto  ParallelPVariant=InternalParameters  IdealPVariant=Disabled  IVariant=InternalParameters  DVariant=InternalParameters  IntegratorVariant=Continuous  SatVariant=Disabled  AWVariant=Passthrough  PCopyVariant=Disabled  TRVariant=Disabled  FdbkBlocksVariant=Forward  IdealPFdbkVariant=Disabled  SatFdbkVariant=Disabled  DerivativeFilterVariant=ContFilter  NVariant=InternalParameters  NCopyVariant=Disabled  FilterICVariant=InternalICsFilter  IntegratorICVariant=InternalICs  ExternalResetVariant=Disabled  TRSumVariant=Passthrough  SumFdbkVariant=Disabled  SumVariant=Sum_PID  TsampFilterVariant=InternalTs  TsampNgainVariant=Passthrough  TsampIntegralVariant=Passthrough  ExternalSaturationOutDataTypeStr=Inherit: Same as second input
  PS-Simulink Converter : nesl_utility/PS-Simulink Converter  PhysicalDomain=network_engine_domain  SubClassName=ps_output  LeftPortType=input  RightPortType=output  PseudoPeriodic=off  Frequencies=[]  Unit=inherit  AffineConversion=off
      settings: SourceProductBaseCode=PW,SS
  PS-Simulink Converter1 : nesl_utility/PS-Simulink Converter  PhysicalDomain=network_engine_domain  SubClassName=ps_output  LeftPortType=input  RightPortType=output  PseudoPeriodic=off  Frequencies=[]  Unit=1  AffineConversion=off
      settings: SourceProductBaseCode=PW,SS
  PS-Simulink Converter2 : nesl_utility/PS-Simulink Converter  PhysicalDomain=network_engine_domain  SubClassName=ps_output  LeftPortType=input  RightPortType=output  PseudoPeriodic=off  Frequencies=[]  Unit=inherit  AffineConversion=off
      settings: SourceProductBaseCode=PW,SS
  PS-Simulink Converter3 : nesl_utility/PS-Simulink Converter  PhysicalDomain=network_engine_domain  SubClassName=ps_output  LeftPortType=input  RightPortType=output  PseudoPeriodic=off  Frequencies=[]  Unit=1  AffineConversion=off
      settings: SourceProductBaseCode=PW,SS
  Scope : Scope
  Scope1 : Scope
  Scope2 : Scope
  Simulink-PS Converter : nesl_utility/Simulink-PS Converter  PhysicalDomain=network_engine_domain  SubClassName=ps_input  LeftPortType=input  RightPortType=output  PseudoPeriodic=off  Frequencies=[]  NoiseDistribution=none  NoiseParameters=[]  Unit=1  AffineConversion=off  FilteringAndDerivatives=provide  SimscapeFilterOrder=1  InputFilterTimeConstant=0.001  UdotUserProvided=0
      settings: SourceProductBaseCode=PW,SS
  Sum : Sum  Inputs=|+-
  Conn1 : PMIOPort  Side=Left
  Conn2 : PMIOPort  Port=2  Side=Right
  q : PMIOPort  Port=3  Side=Left
  meas : Outport
  Outport : Outport  Port=2
  Outport2 : Outport  Port=3
  wires:
  Bus Creator/1 -> meas/1
  PS-Simulink Converter3/1 -> Bus Creator/1  "angleRFknee"
  PS-Simulink Converter1/1 -> Outport/1, Bus Creator/2  "speedRFknee"
  Sum/1 -> Scope1/1, PID Controller/1
  PID Controller/1 -> Bus Creator/3, Simulink-PS Converter/1, Scope/1  "torqueRFknee"
  PS-Simulink Converter2/1 -> Outport2/1
  tddRF_knee/1 -> Scope2/1
  t2ddknee/1 -> Sum/1
  PS-Simulink Converter/1 -> Sum/2
  connections:
  Knee joint/RConn2 -- q/RConn1 -- PS-Simulink Converter3/LConn1
  Knee joint/LConn1 -- Conn1/RConn1
  Conn2/RConn1 -- Knee joint/RConn1
  Knee joint/RConn3 -- PS-Simulink Converter1/LConn1
  Simulink-PS Converter/RConn1 -- Knee joint/LConn2
  PS-Simulink Converter2/LConn1 -- Knee joint/RConn4 -- PS-Simulink Converter/LConn1

== system final_quadruped_210522/Model/Right Leg Front /Measuring Component ==
  Fn : Inport
  Hip : Inport  Port=2
  Fr : Inport  Port=3
  Knee : Inport  Port=4
  Ankle : Inport  Port=5
  Bus Creator : BusCreator  Inputs=9
  Bus Selector : BusSelector  OutputSignals=angleRFknee,speedRFknee,torqueRFknee
  Bus Selector1 : BusSelector  OutputSignals=angleRFhip,speedRFhip,torqueRFhip
  Meas : Outport  VectorParamsAs1DForOutWhenUnconnected=off
  wires:
  Ankle/1 -> Bus Creator/3
  Hip/1 -> Bus Selector1/1
  Fn/1 -> Bus Creator/1
  Bus Creator/1 -> Meas/1
  Fr/1 -> Bus Creator/2
  Knee/1 -> Bus Selector/1
  Bus Selector1/3 -> Bus Creator/7  "<torqueRFhip>"
  Bus Selector1/1 -> Bus Creator/8  "<angleRFhip>"
  Bus Selector1/2 -> Bus Creator/9  "<speedRFhip>"
  Bus Selector/2 -> Bus Creator/4  "<speedRFknee>"
  Bus Selector/3 -> Bus Creator/6  "<torqueRFknee>"
  Bus Selector/1 -> Bus Creator/5  "<angleRFknee>"

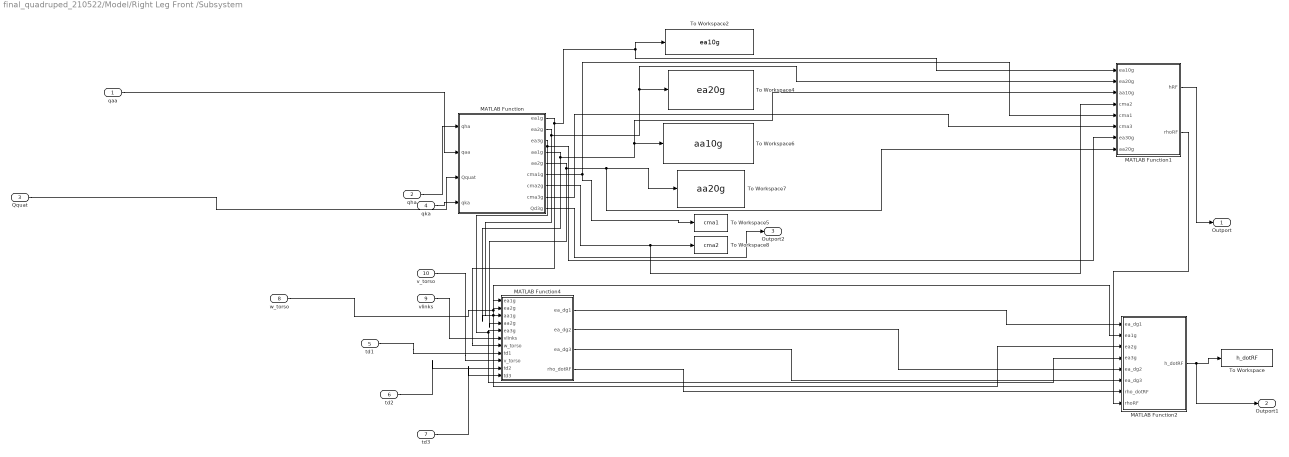
== system final_quadruped_210522/Model/Right Leg Front /Subsystem ==
  qaa : Inport
  qha : Inport  Port=2
  Qquat : Inport  Port=3
  qka : Inport  Port=4
  td1 : Inport  Port=5
  td2 : Inport  Port=6
  td3 : Inport  Port=7
  w_torso : Inport  Port=8
  vlinks : Inport  Port=9
  v_torso : Inport  Port=10
  MATLAB Function : MATLAB Function  TreatAsAtomicUnit=on
  MATLAB Function1 : MATLAB Function  TreatAsAtomicUnit=on
  MATLAB Function2 : MATLAB Function  TreatAsAtomicUnit=on
  MATLAB Function4 : MATLAB Function  TreatAsAtomicUnit=on
  To Workspace : ToWorkspace  VariableName=h_dotRF  SaveFormat=Timeseries  SampleTime=-1
  To Workspace2 : ToWorkspace  VariableName=ea10g  SaveFormat=Timeseries  SampleTime=-1
  To Workspace4 : ToWorkspace  VariableName=ea20g  SaveFormat=Timeseries  SampleTime=-1
  To Workspace5 : ToWorkspace  VariableName=cma1  SaveFormat=Timeseries  SampleTime=-1
  To Workspace6 : ToWorkspace  VariableName=aa10g  SaveFormat=Timeseries  SampleTime=-1
  To Workspace7 : ToWorkspace  VariableName=aa20g  SaveFormat=Timeseries  SampleTime=-1
  To Workspace8 : ToWorkspace  VariableName=cma2  SaveFormat=Timeseries  SampleTime=-1
  Outport : Outport
  Outport1 : Outport  Port=2
  Outport2 : Outport  Port=3
  wires:
  MATLAB Function/8(cma3g) -> MATLAB Function1/6(cma3)
  MATLAB Function/4(aa1g) -> MATLAB Function4/3(aa1g), To Workspace6/1, MATLAB Function1/3(aa10g)
  MATLAB Function/5(aa2g) -> MATLAB Function4/4(aa2g), MATLAB Function1/8(aa20g), To Workspace7/1
  MATLAB Function/1(ea1g) -> To Workspace2/1, MATLAB Function1/1(ea10g), MATLAB Function4/7(w_torso)
  MATLAB Function/7(cma2g) -> MATLAB Function1/4(cma2), To Workspace8/1
  MATLAB Function/3(ea3g) -> MATLAB Function1/7(ea30g), MATLAB Function2/4(ea3g), MATLAB Function4/5(ea3g)
  MATLAB Function/6(cma1g) -> To Workspace5/1, MATLAB Function1/5(cma1)
  MATLAB Function/2(ea2g) -> MATLAB Function1/2(ea20g), To Workspace4/1, MATLAB Function2/3(ea2g), MATLAB Function4/2(ea2g)
  MATLAB Function1/1(hRF) -> Outport/1
  qka/1 -> MATLAB Function/4(qka)
  qaa/1 -> MATLAB Function/2(qaa)
  Qquat/1 -> MATLAB Function/3(Qquat)
  qha/1 -> MATLAB Function/1(qha)
  w_torso/1 -> MATLAB Function2/2(ea1g), MATLAB Function4/1(ea1g)
  td1/1 -> MATLAB Function4/8(td1)
  td2/1 -> MATLAB Function4/10(td2)
  td3/1 -> MATLAB Function4/11(td3)
  vlinks/1 -> MATLAB Function4/6(vlinks)
  v_torso/1 -> MATLAB Function4/9(v_torso)
  MATLAB Function4/1(ea_dg1) -> MATLAB Function2/1(ea_dg1)
  MATLAB Function4/2(ea_dg2) -> MATLAB Function2/5(ea_dg2)
  MATLAB Function4/3(ea_dg3) -> MATLAB Function2/6(ea_dg3)
  MATLAB Function4/4(rho_dotRF) -> MATLAB Function2/7(rho_dotRF)
  MATLAB Function1/2(rhoRF) -> MATLAB Function2/8(rhoRF)
  MATLAB Function2/1(h_dotRF) -> Outport1/1, To Workspace/1
  MATLAB Function/9(Qd3g) -> Outport2/1

== matlab function final_quadruped_210522/Model/Left Leg Front/Subsystem/MATLAB Function ==
  data: eb1g output; eb2g output; eb3g output; qhb input; qab input; Qquat input; qkb input; ab1g output; ab2g output; cmb1g output; cmb2g output; cmb3g output
function [eb1g,eb2g,eb3g,ab1g,ab2g,cmb1g,cmb2g,cmb3g] = fcn(qhb,qab,Qquat,qkb)
%%
lower_leg_length = 10;
upper_leg_length = 10;
foot_offset=[-1; 0; 0];

%%
Qd10=zeros(3,3);
% disp(Qquat);
% Qquat=reshape(Qquat,4,1);
Qquat;
Qd0g=quat2rotm([Qquat(1) Qquat(2) Qquat(3) Qquat(4)]);
% Qd0geul=quat2eul(Qquat);
% Qd0g=eul2rotm(Qd0geul);
Qd10=[cos(qhb) 0 sin(qhb);
      0 1 0 ;
      -sin(qhb) 0 cos(qhb)];
Qd1g=Qd10*Qd0g;
  
Qd21=[cos(qkb) 0 sin(qkb);
      0 1 0 ;
      -sin(qkb) 0 cos(qkb)];
  
Qd32=[1 0 0;
      0 cos(qab) -sin(qab);
      0 sin(qab) cos(qab)];
  
Qd20 = Qd21* Qd10;
Qd30=Qd32*Qd20;
Qd2g=Qd20*Qd0g;
Qd3g=Qd30*Qd0g;

%axis in local frames
ed1l=[0;
      1;
      0];
ed2l=[0;
      1;
      0];
ed3l=[0;
     0;
     1];
  
%link vector in local frame
ad1l=[0;
      0;
      -upper_leg_length];
   
ad2l=[0;
      0;
      -lower_leg_length];
         
%axis in global frames
eb1g = Qd1g*ed1l;
eb2g = Qd2g*ed2l;
eb3g = Qd3g*ed3l;

%link vector in global frame
ab1g = Qd1g*ad1l;
ab2g = Qd2g*ad2l;

%COM distances in base frame
cmb1g=ab1g/2;
cmb2g=ab2g/2;
cmb3g=Qd3g*foot_offset;


end

== matlab function final_quadruped_210522/Model/Right Leg Back/Subsystem/MATLAB Function ==
  data: ec1g output; ec2g output; ec3g output; qhc input; qac input; Qquat input; qkc input; ac1g output; ac2g output; cmc1g output; cmc2g output; cmc3g output
function [ec1g,ec2g,ec3g,ac1g,ac2g,cmc1g,cmc2g,cmc3g] = fcn(qhc,qac,Qquat,qkc)
%%
lower_leg_length = 10;
upper_leg_length = 10;
foot_offset=[-1; 0; 0];

%%
Qd0g=quat2rotm([Qquat(1) Qquat(2) Qquat(3) Qquat(4)]);
Qd10=[cos(qhc) 0 sin(qhc);
      0 1 0 ;
      -sin(qhc) 0 cos(qhc)];
Qd1g=Qd10*Qd0g;
  
Qd21=[cos(qkc) 0 sin(qkc);
      0 1 0 ;
      -sin(qkc) 0 cos(qkc)];
  
Qd32=[1 0 0;
      0 cos(qac) -sin(qac);
      0 sin(qac) cos(qac)];
  
Qd20 = Qd21* Qd10;
Qd30=Qd32*Qd20;
Qd2g=Qd20*Qd0g;
Qd3g=Qd30*Qd0g;

%axis in local frames
ed1l=[0;
      1;
      0];
ed2l=[0;
      1;
      0];
ed3l=[0;
     0;
     1];
  
%link vector in local frame
ad1l=[0;
      0;
      -upper_leg_length];
   
ad2l=[0;
      0;
      -lower_leg_length];
         
%axis in global frames
ec1g = Qd1g*ed1l;
ec2g = Qd2g*ed2l;
ec3g = Qd3g*ed3l;

%link vector in global frame
ac1g = Qd1g*ad1l;
ac2g = Qd2g*ad2l;

%COM distances in base frame
cmc1g=ac1g/2;
cmc2g=ac2g/2;
cmc3g=Qd3g*foot_offset;


end

== matlab function final_quadruped_210522/Model/Left LegBack/Subsystem/MATLAB Function ==
  data: ed1g output; ed2g output; ed3g output; qhd input; qad input; Qquat input; qkd input; ad1g output; ad2g output; cmd1g output; cmd2g output; cmd3g output
function [ed1g,ed2g,ed3g,ad1g,ad2g,cmd1g,cmd2g,cmd3g] = fcn(qhd,qad,Qquat, qkd)
%%
lower_leg_length = 10;
upper_leg_length = 10;
foot_offset=[-1; 0; 0];

%%
Qd0g=quat2rotm([Qquat(1) Qquat(2) Qquat(3) Qquat(4)]);
Qd10=[cos(qhd) 0 sin(qhd);
      0 1 0 ;
      -sin(qhd) 0 cos(qhd)];
Qd1g=Qd10*Qd0g;
  
Qd21=[cos(qkd) 0 sin(qkd);
      0 1 0 ;
      -sin(qkd) 0 cos(qkd)];
  
Qd32=[1 0 0;
      0 cos(qad) -sin(qad);
      0 sin(qad) cos(qad)];
  
Qd20 = Qd21* Qd10;
Qd30=Qd32*Qd20;
Qd2g=Qd20*Qd0g;
Qd3g=Qd30*Qd0g;

%axis in local frames
ed1l=[0;
      1;
      0];
ed2l=[0;
      1;
      0];
ed3l=[0;
     0;
     1];
  
%link vector in local frame
ad1l=[0;
      0;
      -upper_leg_length];
   
ad2l=[0;
      0;
      -lower_leg_length];
         
%axis in global frames
ed1g = Qd1g*ed1l;
ed2g = Qd2g*ed2l;
ed3g = Qd3g*ed3l;

%link vector in global frame
ad1g = Qd1g*ad1l;
ad2g = Qd2g*ad2l;

%COM distances in base frame
cmd1g=ad1g/2;
cmd2g=ad2g/2;
cmd3g=Qd3g*foot_offset;


end

== matlab function final_quadruped_210522/Model/MATLAB Function4 ==
  data: hLF input; hRB input; hLB input; h_dotLF input; hRF input; h_dotRF input; tddRF output; v_torso input; tddLF output; tddRB output; tddLB output; h output; h_dot output; h_dotRB input; h_dotLB input; theta_d_des output; M output
function [tddRF,tddLF,tddRB,tddLB,h,h_dot,theta_d_des,M] = fcn(hLF, hRB, hLB, h_dotLF, hRF,h_dotRF, v_torso, h_dotRB, h_dotLB)
%%
lower_leg_length = 10;
upper_leg_length = 10;
density = 1000;
foot_density=2000;
leg_radius = 0.75;
foot_x = 8;
foot_y = 6;
foot_z = 1;
torso_y = 16;
torso_x = 25;
torso_z = 10;
m_ul=density*leg_radius*leg_radius*upper_leg_length*3.141592653589*0.01*0.01*0.01;
m_ll=density*leg_radius*leg_radius*lower_leg_length*3.141592653589*0.01*0.01*0.01;
m_foot=foot_density*foot_x*foot_y*foot_z*0.000001;
m_torso=density*torso_x*torso_y*torso_z*0.000001;
M=m_torso+(4*(m_ul+m_ll+m_foot));
%%
h=[hRF hLF hRB hLB];
h_dot=[h_dotRF h_dotLF h_dotRB h_dotLB];
theta_d_des=M*(-pinv(h)*v_torso);

tddRF_hip=theta_d_des(1);
tddRF_knee=theta_d_des(2);
tddRF_ankle=theta_d_des(3);
tddLF_hip=theta_d_des(4);
tddLF_knee=theta_d_des(5);
tddLF_ankle=theta_d_des(6);
tddRB_hip=theta_d_des(7);
tddRB_knee=theta_d_des(8);
tddRB_ankle=theta_d_des(9);
tddLB_hip=theta_d_des(10);
tddLB_knee=theta_d_des(11);
tddLB_ankle=theta_d_des(12);

tddRF=[tddRF_hip tddRF_knee tddRF_ankle];
tddLF=[tddLF_hip tddLF_knee tddLF_ankle];
tddRB=[tddRB_hip tddRB_knee tddRB_ankle];
tddLB=[tddLB_hip tddLB_knee tddLB_ankle];
end

== matlab function final_quadruped_210522/Model/Right Leg Front /Subsystem/MATLAB Function1 ==
  data: ea10g input; ea20g input; aa10g input; cma2 input; cma1 input; cma3 input; ea30g input; aa20g input; hRF output; rhoRF output
function [hRF,rhoRF] = fcn(ea10g, ea20g, aa10g, cma2, cma1, cma3, ea30g, aa20g)
%%
lower_leg_length = 10;
upper_leg_length = 10;
density = 1000;
foot_density=2000;
leg_radius = 0.75;
foot_x = 8;
foot_y = 6;
foot_z = 1;
m_ul=density*leg_radius*leg_radius*upper_leg_length*3.141592653589*0.01*0.01*0.01;
m_ll=density*leg_radius*leg_radius*lower_leg_length*3.141592653589*0.01*0.01*0.01;
m_foot=foot_density*foot_x*foot_y*foot_z*0.000001;
%%
scf=zeros(3,3);
sof=zeros(3,3);
rhoRF=zeros(3,3,3);
scf(:,1)=cma1;
scf(:,2)=aa10g+cma2;
scf(:,3)=aa10g+aa20g+cma3;
sof(:,1)=[0;0;0];
sof(:,2)=aa10g;
sof(:,3)=aa10g+aa20g;
for i=1:3
    for j=1:3
        if j<i
rhoRF(:,j,i)=zeros(3,1);
        else
rhoRF(:,j,i)=scf(:,j)-sof(:,i);
        end
    end
end
h1=(m_ul*cross(ea10g,rhoRF(:,1,1)))+(m_ll*cross(ea10g,rhoRF(:,2,1)))+(m_foot*cross(ea10g,rhoRF(:,3,1)));
h2=(m_ll*cross(ea20g,rhoRF(:,2,2)))+(m_foot*cross(ea20g,rhoRF(:,3,2)));
h3=m_foot*(cross(ea30g,rhoRF(:,3,3)));

hRF =[h1 h2 h3];



end

== matlab function final_quadruped_210522/Model/Left Leg Front/Subsystem/MATLAB Function1 ==
  data: eb10g input; eb20g input; ab10g input; cmb2 input; cmb1 input; cmb3 input; eb30g input; hLF output; ab20g input; rhoLF output
function [hLF,rhoLF] = fcn(eb10g, eb20g, ab10g, cmb2, cmb1, cmb3, eb30g, ab20g)
%%
lower_leg_length = 10;
upper_leg_length = 10;
density = 1000;
foot_density=2000;
leg_radius = 0.75;
foot_x = 8;
foot_y = 6;
foot_z = 1;
m_ul=density*leg_radius*leg_radius*upper_leg_length*3.141592653589*0.01*0.01*0.01;
m_ll=density*leg_radius*leg_radius*lower_leg_length*3.141592653589*0.01*0.01*0.01;
m_foot=foot_density*foot_x*foot_y*foot_z*0.000001;
%%
scf=zeros(3,3);
sof=zeros(3,3);
rhoLF=zeros(3,3,3);
scf(:,1)=cmb1;
scf(:,2)=ab10g+cmb2;
scf(:,3)=ab10g+ab20g+cmb3;
sof(:,1)=[0;0;0];
sof(:,2)=ab10g;
sof(:,3)=ab10g+ab20g;
for i=1:3
    for j=1:3
        if j<i
rhoLF(:,j,i)=zeros(3,1);
        else
rhoLF(:,j,i)=scf(:,j)-sof(:,i);
        end
    end
end
h1=(m_ul*cross(eb10g,rhoLF(:,1,1)))+(m_ll*cross(eb10g,rhoLF(:,2,1)))+(m_foot*cross(eb10g,rhoLF(:,3,1)));
h2=(m_ll*cross(eb20g,rhoLF(:,2,2)))+(m_foot*cross(eb20g,rhoLF(:,3,2)));
h3=m_foot*(cross(eb30g,rhoLF(:,3,3)));

hLF =[h1 h2 h3];



end

== matlab function final_quadruped_210522/Model/Right Leg Back/Subsystem/MATLAB Function1 ==
  data: ec10g input; ec20g input; ac10g input; cmc2 input; cmc1 input; cmc3 input; ec30g input; ac20g input; hRB output; rhoRB output
function [hRB,rhoRB] = fcn(ec10g, ec20g, ac10g, cmc2, cmc1, cmc3, ec30g, ac20g)
%%
lower_leg_length = 10;
upper_leg_length = 10;
density = 1000;
foot_density=2000;
leg_radius = 0.75;
foot_x = 8;
foot_y = 6;
foot_z = 1;
m_ul=density*leg_radius*leg_radius*upper_leg_length*3.141592653589*0.01*0.01*0.01;
m_ll=density*leg_radius*leg_radius*lower_leg_length*3.141592653589*0.01*0.01*0.01;
m_foot=foot_density*foot_x*foot_y*foot_z*0.000001;
%%
scf=zeros(3,3);
sof=zeros(3,3);
rhoRB=zeros(3,3,3);
scf(:,1)=cmc1;
scf(:,2)=ac10g+cmc2;
scf(:,3)=ac10g+ac20g+cmc3;
sof(:,1)=[0;0;0];
sof(:,2)=ac10g;
sof(:,3)=ac10g+ac20g;
for i=1:3
    for j=1:3
        if j<i
rhoRB(:,j,i)=zeros(3,1);
        else
rhoRB(:,j,i)=scf(:,j)-sof(:,i);
        end
    end
end
h1=(m_ul*cross(ec10g,rhoRB(:,1,1)))+(m_ll*cross(ec10g,rhoRB(:,2,1)))+(m_foot*cross(ec10g,rhoRB(:,3,1)));
h2=(m_ll*cross(ec20g,rhoRB(:,2,2)))+(m_foot*cross(ec20g,rhoRB(:,3,2)));
h3=m_foot*(cross(ec30g,rhoRB(:,3,3)));

hRB =[h1 h2 h3];



end
